simulink model "sine_sim"  (R2018a)
settings: Solver=VariableStepAuto  StartTime=0.0  StopTime=10.0  RelTol=1e-3
settings Model: Creator=Li Gen  LastModifiedBy=Li Gen

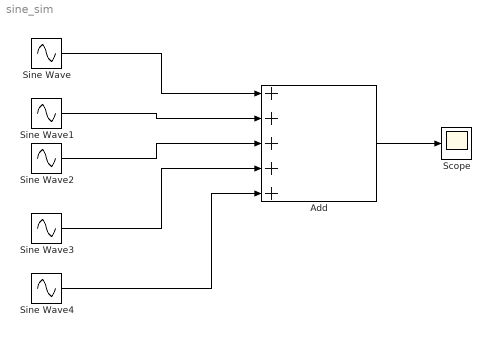
== system sine_sim ==
  Add : Sum  Inputs=+++++
  Scope : Scope
  Sine Wave : Sin  Frequency=2*pi  SampleTime=0
  Sine Wave1 : Sin  Amplitude=1/3  Frequency=6*pi  SampleTime=0
  Sine Wave2 : Sin  Amplitude=1/5  Frequency=10*pi  SampleTime=0
  Sine Wave3 : Sin  Amplitude=1/7  Frequency=14*pi  SampleTime=0
  Sine Wave4 : Sin  Amplitude=1/9  Frequency=18*pi  SampleTime=0
  wires:
  Sine Wave/1 -> Add/1
  Sine Wave1/1 -> Add/2
  Sine Wave2/1 -> Add/3
  Sine Wave3/1 -> Add/4
  Sine Wave4/1 -> Add/5
  Add/1 -> Scope/1
